simulink model "psm_stromregelung_done"  (R2025a)
settings: Solver=ode45  StartTime=0.0  StopTime=1.5  MaxStep=1e-4  RelTol=1e-3
values from neighbouring files (symbols this model uses):
  L = 0.01    [build_stromregelung.m]
  R = 1.0    (= 1)    [build_stromregelung.m]
  Udc = 30    [build_stromregelung.m]
libraries: slpidlib x1
settings Model: Creator=moham  LastModifiedBy=moham
settings SolverCC: MaxConsecutiveZCs=10000  ZeroCrossAlgorithm=Adaptive

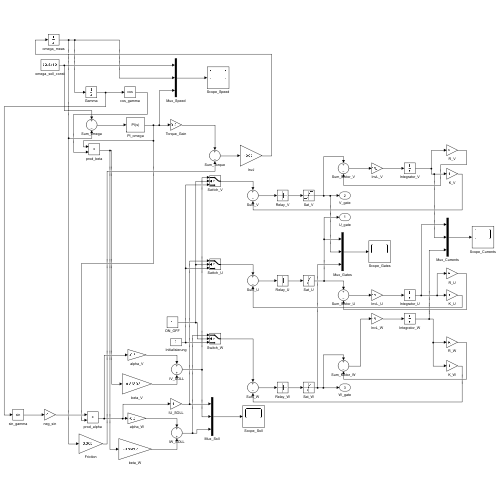
[thumbnail: Simulink's stored preview of the top-level diagram]
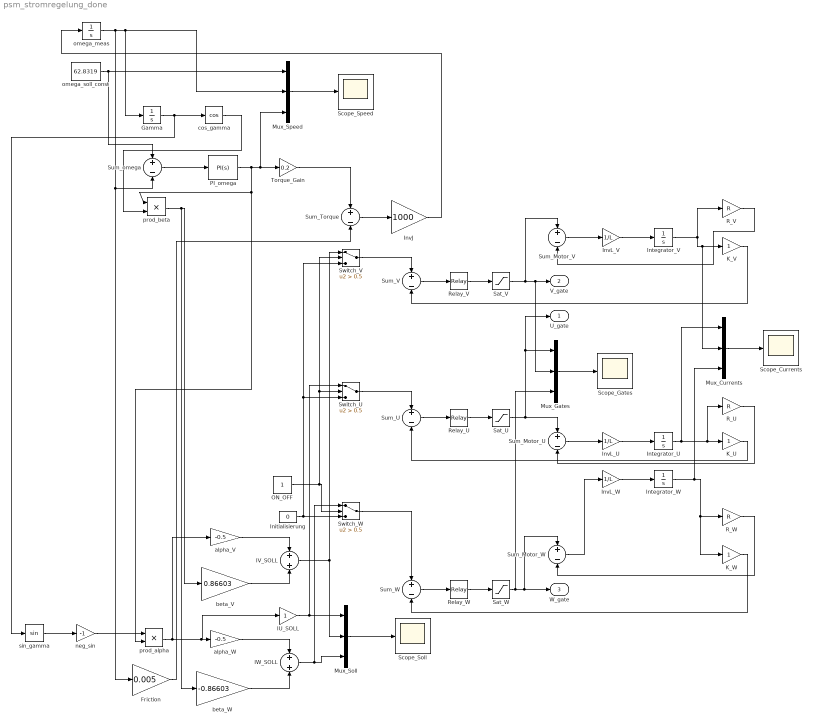
== system psm_stromregelung_done ==
  Friction : Gain  Gain=0.005
  Gamma : Integrator
  IU_SOLL : Gain
  IV_SOLL : Sum
  IW_SOLL : Sum
  Initialisierung : Constant  Value=0
  Integrator_U : Integrator
  Integrator_V : Integrator
  Integrator_W : Integrator
  InvJ : Gain  Gain=1000
  InvL_U : Gain  Gain=1/L
  InvL_V : Gain  Gain=1/L
  InvL_W : Gain  Gain=1/L
  K_U : Gain
  K_V : Gain
  K_W : Gain
  Mux_Currents : Mux  Inputs=3
  Mux_Gates : Mux  Inputs=3
  Mux_Soll : Mux  Inputs=3
  Mux_Speed : Mux  Inputs=3
  ON_OFF : Constant
  PI_omega : slpidlib/PID Controller  Controller=PI  Form=Parallel  TimeDomain=Continuous-time  UseExternalTs=off  SampleTime=-1  IntegratorMethod=Forward Euler  FilterMethod=Forward Euler  ControllerParametersSource=internal  P=0.02  I=1  UseKiTs=off  D=0  UseExternalDerivativeSource=off  N=100  UseFilter=on  TunerSelectOption=Transfer Function Based (PID Tuner App)  InitialConditionSource=internal  InitialConditionForIntegrator=0  InitialConditionForFilter=0  DifferentiatorICPrevScaledInput=0  ExternalReset=none  TrackingMode=off  Kt=1  LimitOutput=off  SatLimitsSource=internal  UpperSaturationLimit=3  LowerSaturationLimit=-3  LinearizeAsGain=on  AntiWindupMode=none  Kb=1  LimitIntegrator=off  UpperIntegratorSaturationLimit=inf  LowerIntegratorSaturationLimit=-inf  POutMin=[]  POutMax=[]  IOutMin=[]  IOutMax=[]  DOutMin=[]  DOutMax=[]  NOutMin=[]  NOutMax=[]  SumOutMin=[]  SumOutMax=[]  SaturationOutMin=[]  SaturationOutMax=[]  PParamMin=[]  PParamMax=[]  IParamMin=[]  IParamMax=[]  DParamMin=[]  DParamMax=[]  NParamMin=[]  NParamMax=[]  KbParamMin=[]  KbParamMax=[]  KtParamMin=[]  KtParamMax=[]  KbOutMin=[]  KbOutMax=[]  KtOutMin=[]  KtOutMax=[]  IntegratorOutMin=[]  IntegratorOutMax=[]  FilterOutMin=[]  FilterOutMax=[]  SumI1OutMin=[]  SumI1OutMax=[]  SumI2OutMin=[]  SumI2OutMax=[]  SumI3OutMin=[]  SumI3OutMax=[]  SumI4OutMin=[]  SumI4OutMax=[]  SumDOutMin=[]  SumDOutMax=[]  DifferentiatorOutMin=[]  DifferentiatorOutMax=[]  FilterDiffOutCoefMin=[]  FilterDiffOutCoefMax=[]  ReciprocalOutMin=[]  ReciprocalOutMax=[]  SumDenOutMin=[]  SumDenOutMax=[]  SumNumOutMin=[]  SumNumOutMax=[]  DivideOutMin=[]  DivideOutMax=[]  UdiffTsProdOutMin=[]  UdiffTsProdOutMax=[]  NTsProdOutMin=[]  NTsProdOutMax=[]  UintegralTsProdOutMin=[]  UintegralTsProdOutMax=[]  UngainTsProdOutMin=[]  UngainTsProdOutMax=[]  ClampingZeroOutDataTypeStr=Inherit: Inherit via back propagation  ClampingZeroOutMin=[]  ClampingZeroOutMax=[]  FilterDenConstantOutDataTypeStr=Inherit: Inherit via back propagation  FilterDenConstantOutMin=[]  FilterDenConstantOutMax=[]  PCopyOutDataTypeStr=Inherit: Inherit via back propagation  PCopyOutMin=[]  PCopyOutMax=[]  NCopyOutDataTypeStr=Inherit: Inherit via back propagation  NCopyOutMin=[]  NCopyOutMax=[]  IntegratorContinuousStateAttributes=''  IntegratorStateMustResolveToSignalObject=off  IntegratorRTWStateStorageClass=Auto  FilterContinuousStateAttributes=''  FilterStateMustResolveToSignalObject=off  FilterRTWStateStorageClass=Auto  ParallelPVariant=InternalParameters  IdealPVariant=Disabled  IVariant=InternalParameters  DVariant=Disabled  IntegratorVariant=Continuous  SatVariant=Disabled  AWVariant=Passthrough  PCopyVariant=Disabled  TRVariant=Disabled  FdbkBlocksVariant=Forward  IdealPFdbkVariant=Disabled  SatFdbkVariant=Disabled  DerivativeFilterVariant=Disabled  NVariant=Disabled  NCopyVariant=Disabled_SignalSpec  FilterICVariant=Disabled  IntegratorICVariant=InternalICs  ExternalResetVariant=Disabled  TRSumVariant=Passthrough  SumFdbkVariant=Disabled  SumVariant=Sum_PI  TsampFilterVariant=InternalTs  TsampNgainVariant=Passthrough  TsampIntegralVariant=Disabled_SignalSpec  ExternalSaturationOutDataTypeStr=Inherit: Same as second input  DerivativeSourceVariant=Disabled  PreIntVariant=InternalPreInt
  R_U : Gain  Gain=R
  R_V : Gain  Gain=R
  R_W : Gain  Gain=R
  Relay_U : Relay  OnSwitchValue=0.1  OffSwitchValue=-0.1  OffOutputValue=-1
  Relay_V : Relay  OnSwitchValue=0.1  OffSwitchValue=-0.1  OffOutputValue=-1
  Relay_W : Relay  OnSwitchValue=0.1  OffSwitchValue=-0.1  OffOutputValue=-1
  Sat_U : Saturate  UpperLimit=Udc  LowerLimit=-Udc
  Sat_V : Saturate  UpperLimit=Udc  LowerLimit=-Udc
  Sat_W : Saturate  UpperLimit=Udc  LowerLimit=-Udc
  Scope_Currents : Scope
  Scope_Gates : Scope
  Scope_Soll : Scope
  Scope_Speed : Scope
  Sum_Motor_U : Sum  Inputs=+-
  Sum_Motor_V : Sum  Inputs=+-
  Sum_Motor_W : Sum  Inputs=+-
  Sum_Torque : Sum  Inputs=+-
  Sum_U : Sum  Inputs=+-
  Sum_V : Sum  Inputs=+-
  Sum_W : Sum  Inputs=+-
  Sum_omega : Sum  Inputs=+-
  Switch_U : Switch  Criteria=u2 > Threshold  Threshold=0.5  SaturateOnIntegerOverflow=off  InputSameDT=off
  Switch_V : Switch  Criteria=u2 > Threshold  Threshold=0.5  SaturateOnIntegerOverflow=off  InputSameDT=off
  Switch_W : Switch  Criteria=u2 > Threshold  Threshold=0.5  SaturateOnIntegerOverflow=off  InputSameDT=off
  Torque_Gain : Gain  Gain=0.2
  alpha_V : Gain  Gain=-0.5
  alpha_W : Gain  Gain=-0.5
  beta_V : Gain  Gain=0.86603
  beta_W : Gain  Gain=-0.86603
  cos_gamma : Trigonometry  Operator=cos
  neg_sin : Gain  Gain=-1
  omega_meas : Integrator
  omega_soll_const : Constant  Value=62.8319
  prod_alpha : Product
  prod_beta : Product
  sin_gamma : Trigonometry
  U_gate : Outport
  V_gate : Outport  Port=2
  W_gate : Outport  Port=3
  wires:
  sin_gamma/1 -> neg_sin/1
  InvL_U/1 -> Integrator_U/1
  Initialisierung/1 -> Switch_U/3, Switch_V/3, Switch_W/3
  omega_meas/1 -> Sum_omega/2, Friction/1, Gamma/1, Mux_Speed/2
  Gamma/1 -> sin_gamma/1, cos_gamma/1
  Sum_Motor_U/1 -> InvL_U/1
  Friction/1 -> Sum_Torque/2
  omega_soll_const/1 -> Sum_omega/1, Mux_Speed/1
  Integrator_W/1 -> K_W/1, R_W/1, Mux_Currents/3
  Mux_Speed/1 -> Scope_Speed/1
  prod_alpha/1 -> IU_SOLL/1, alpha_W/1, alpha_V/1
  neg_sin/1 -> prod_alpha/1
  Sum_omega/1 -> PI_omega/1
  prod_beta/1 -> beta_V/1, beta_W/1
  cos_gamma/1 -> prod_beta/2
  Relay_W/1 -> Sat_W/1
  PI_omega/1 -> prod_alpha/2, prod_beta/1, Torque_Gain/1, Mux_Speed/3
  InvL_V/1 -> Integrator_V/1
  alpha_V/1 -> IV_SOLL/1
  Integrator_V/1 -> K_V/1, Mux_Currents/2, R_V/1
  Sat_U/1 -> U_gate/1, Mux_Gates/1, Sum_Motor_U/1
  beta_V/1 -> IV_SOLL/2
  alpha_W/1 -> IW_SOLL/1
  beta_W/1 -> IW_SOLL/2
  Torque_Gain/1 -> Sum_Torque/1
  ON_OFF/1 -> Switch_U/2, Switch_V/2, Switch_W/2
  IV_SOLL/1 -> Switch_V/1, Mux_Soll/2
  Mux_Gates/1 -> Scope_Gates/1
  Sum_Motor_V/1 -> InvL_V/1
  Relay_U/1 -> Sat_U/1
  IU_SOLL/1 -> Switch_U/1, Mux_Soll/1
  IW_SOLL/1 -> Switch_W/1, Mux_Soll/3
  Sum_Torque/1 -> InvJ/1
  K_U/1 -> Sum_U/2
  Switch_V/1 -> Sum_V/1
  InvL_W/1 -> Integrator_W/1
  Switch_U/1 -> Sum_U/1
  Switch_W/1 -> Sum_W/1
  Mux_Soll/1 -> Scope_Soll/1
  K_W/1 -> Sum_W/2
  InvJ/1 -> omega_meas/1
  Sum_V/1 -> Relay_V/1
  Sat_V/1 -> V_gate/1, Mux_Gates/2, Sum_Motor_V/1
  Sum_U/1 -> Relay_U/1
  Sum_W/1 -> Relay_W/1
  Relay_V/1 -> Sat_V/1
  Sat_W/1 -> Sum_Motor_W/1, W_gate/1, Mux_Gates/3
  Sum_Motor_W/1 -> InvL_W/1
  Integrator_U/1 -> K_U/1, R_U/1, Mux_Currents/1
  R_V/1 -> Sum_Motor_V/2
  K_V/1 -> Sum_V/2
  Mux_Currents/1 -> Scope_Currents/1
  R_U/1 -> Sum_Motor_U/2
  R_W/1 -> Sum_Motor_W/2
